simulink library "CBRModel_lib"  (Simulink 10.2)
settings: Solver=ode45  StartTime=0.0  StopTime=10.0  RelTol=1e-3  EnableMultiTasking=on
libraries: ExampleModel_lib x18, powerlib x11, $bdroot x4, powerlib_extras x4
settings Model: RequirementInfo="{}  %GIDa_6317c1c3_1285_46a1_a401_c249d430af69"  Creator=jde1  LastModifiedBy=albert

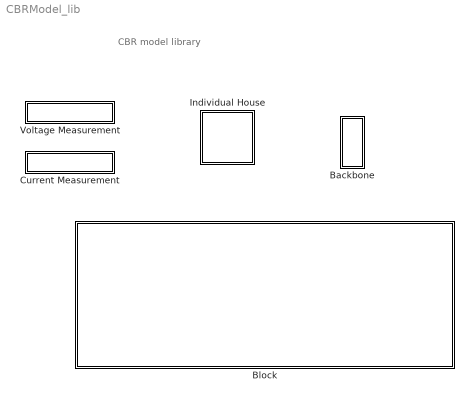
== system CBRModel_lib ==
  note: CBR model library
  Backbone : Subsystem  mask{length=0.0465}
      mask TypeOptions length: line_A/Length | line_B/Length | line_C/Length | line_N/Length
  Block : Subsystem
  Current Measurement : Subsystem  StopFcn=|
      | myname = getfullname(gcb);                                                                      
      | rto = get_param([myname '/RMS Display'], 'RuntimeObject');                                      
      | set_param(myname, 'MaskDisplay', ['color(''blue''); disp(' num2str(rto.InputPort(1).Data) ')']);
      mask Display:
      | port_label('lconn', 1, '+')
      | port_label('rconn', 1, '-')
      | color('blue')
      | disp('0')
  Individual House : Subsystem  mask{length=0.025}
      mask prompts: length "Length of service line (km)"
      mask TypeOptions length: Service Active/Length | Service Neutral/Length
      mask Display:
      | plot([20 30 40 20 20 40 40], [30 40 30 30 10 10 30])
      | port_label('LConn',1,'+')
      | port_label('RConn',1,'-')
  Voltage Measurement : Subsystem  StopFcn=|
      | myname = getfullname(gcb);                                                                      
      | rto = get_param([myname '/RMS Display'], 'RuntimeObject');                                      
      | set_param(myname, 'MaskDisplay', ['color(''blue''); disp(' num2str(rto.InputPort(1).Data) ')']);
      mask Display:
      | port_label('lconn', 1, '+')
      | port_label('rconn', 1, '-')
      | color('blue')
      | disp('0')

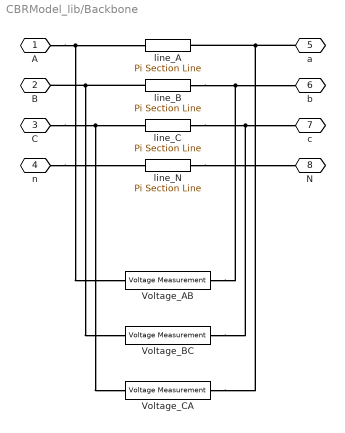
== system CBRModel_lib/Backbone ==
  Voltage_AB : $bdroot/Voltage Measurement  SystemSampleTime=-1  VariantActivationTime=update diagram  Latency=0  AutoFrameSizeCalculation=off
  Voltage_BC : $bdroot/Voltage Measurement  SystemSampleTime=-1  VariantActivationTime=update diagram  Latency=0  AutoFrameSizeCalculation=off
  Voltage_CA : $bdroot/Voltage Measurement  SystemSampleTime=-1  VariantActivationTime=update diagram  Latency=0  AutoFrameSizeCalculation=off
  line_A : powerlib/Elements/Pi Section Line  LConnTagsString=__new0  RConnTagsString=__new0  Phases=1  PiSections=1  Length=length  Frequency=50  Resistance=0.497  Inductance=1.2032e-3  Capacitance=1e-9  Measurements=None  Measurements2=None
      settings: AttributesFormatString=\n  SourceProductBaseCode=PS
  line_B : powerlib/Elements/Pi Section Line  LConnTagsString=__new0  RConnTagsString=__new0  Phases=1  PiSections=1  Length=length  Frequency=50  Resistance=0.497  Inductance=1.2032e-3  Capacitance=1e-9  Measurements=None  Measurements2=None
      settings: AttributesFormatString=\n  SourceProductBaseCode=PS
  line_C : powerlib/Elements/Pi Section Line  LConnTagsString=__new0  RConnTagsString=__new0  Phases=1  PiSections=1  Length=length  Frequency=50  Resistance=0.497  Inductance=1.2032e-3  Capacitance=1e-9  Measurements=None  Measurements2=None
      settings: AttributesFormatString=\n  SourceProductBaseCode=PS
  line_N : powerlib/Elements/Pi Section Line  LConnTagsString=__new0  RConnTagsString=__new0  Phases=1  PiSections=1  Length=length  Frequency=50  Resistance=0.497  Inductance=1.2032e-3  Capacitance=1e-9  Measurements=None  Measurements2=None
      settings: AttributesFormatString=\n  SourceProductBaseCode=PS
  A : PMIOPort  Side=Left
  B : PMIOPort  Port=2  Side=Left
  C : PMIOPort  Port=3  Side=Left
  n : PMIOPort  Port=4  Side=Left
  a : PMIOPort  Port=5  Side=Right
  b : PMIOPort  Port=6  Side=Right
  c : PMIOPort  Port=7  Side=Right
  N : PMIOPort  Port=8  Side=Right
  connections:
  n/RConn1 -- line_N/RConn1
  line_N/LConn1 -- N/RConn1
  a/RConn1 -- line_A/RConn1 -- Voltage_CA/RConn1
  line_B/RConn1 -- b/RConn1 -- Voltage_AB/RConn1
  line_C/RConn1 -- c/RConn1 -- Voltage_BC/RConn1
  C/RConn1 -- line_C/LConn1 -- Voltage_CA/LConn1
  line_B/LConn1 -- B/RConn1 -- Voltage_BC/LConn1
  A/RConn1 -- line_A/LConn1 -- Voltage_AB/LConn1

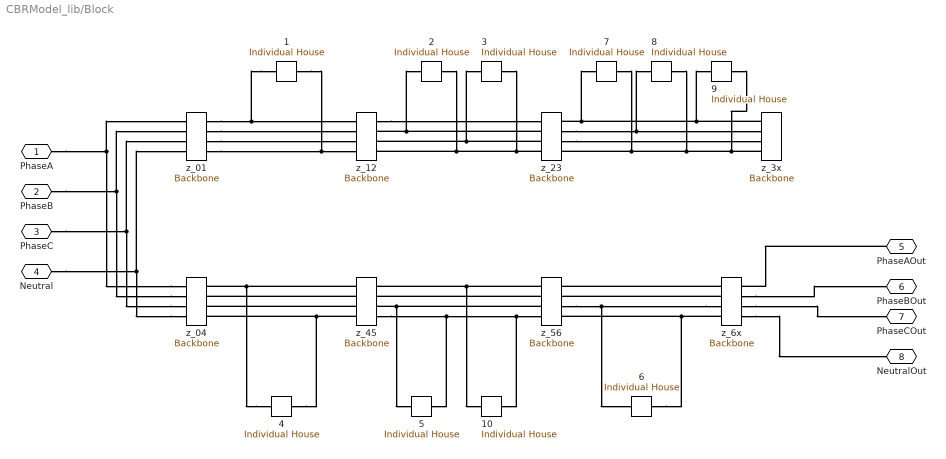
== system CBRModel_lib/Block ==
  {1..10} (10 alike) : ExampleModel_lib/Individual House  length=0.025
  z_01 : ExampleModel_lib/Backbone  length=0.02
  z_04 : ExampleModel_lib/Backbone  length=0.02
  z_{12,23,45,56} (4 alike) : ExampleModel_lib/Backbone  length=0.02
  z_3x : ExampleModel_lib/Backbone  length=0.02
  z_6x : ExampleModel_lib/Backbone  length=0.02
  PhaseA : PMIOPort  Side=Left
  PhaseB : PMIOPort  Port=2  Side=Left
  PhaseC : PMIOPort  Port=3  Side=Left
  Neutral : PMIOPort  Port=4  Side=Left
  PhaseAOut : PMIOPort  Port=5  Side=Right
  PhaseBOut : PMIOPort  Port=6  Side=Right
  PhaseCOut : PMIOPort  Port=7  Side=Right
  NeutralOut : PMIOPort  Port=8  Side=Right
  connections:
  3/LConn1 -- z_23/LConn3 -- z_12/RConn3
  10/RConn1 -- z_45/RConn4 -- 5/RConn1 -- z_56/LConn4
  z_04/LConn3 -- PhaseC/RConn1 -- z_01/LConn3
  z_04/LConn2 -- PhaseB/RConn1 -- z_01/LConn2
  7/RConn1 -- z_3x/LConn4 -- 9/RConn1 -- 8/RConn1 -- z_23/RConn4
  8/LConn1 -- z_23/RConn2 -- z_3x/LConn2
  2/RConn1 -- z_23/LConn4 -- 3/RConn1 -- z_12/RConn4
  4/RConn1 -- z_45/LConn4 -- z_04/RConn4
  7/LConn1 -- z_3x/LConn1 -- 9/LConn1 -- z_23/RConn1
  10/LConn1 -- z_56/LConn1 -- z_45/RConn1
  1/RConn1 -- z_12/LConn4 -- z_01/RConn4
  z_6x/LConn4 -- z_56/RConn4 -- 6/RConn1
  z_6x/LConn3 -- z_56/RConn3 -- 6/LConn1
  z_04/LConn1 -- PhaseA/RConn1 -- z_01/LConn1
  1/LConn1 -- z_12/LConn1 -- z_01/RConn1
  4/LConn1 -- z_45/LConn1 -- z_04/RConn1
  z_04/LConn4 -- Neutral/RConn1 -- z_01/LConn4
  5/LConn1 -- z_56/LConn3 -- z_45/RConn3
  2/LConn1 -- z_23/LConn2 -- z_12/RConn2
  PhaseAOut/RConn1 -- z_6x/RConn1
  z_56/LConn2 -- z_45/RConn2
  z_45/LConn2 -- z_04/RConn2
  z_01/RConn2 -- z_12/LConn2
  z_45/LConn3 -- z_04/RConn3
  z_6x/LConn1 -- z_56/RConn1
  z_01/RConn3 -- z_12/LConn3
  z_12/RConn1 -- z_23/LConn1
  z_23/RConn3 -- z_3x/LConn3
  z_6x/LConn2 -- z_56/RConn2
  z_6x/RConn4 -- NeutralOut/RConn1
  z_6x/RConn2 -- PhaseBOut/RConn1
  z_6x/RConn3 -- PhaseCOut/RConn1

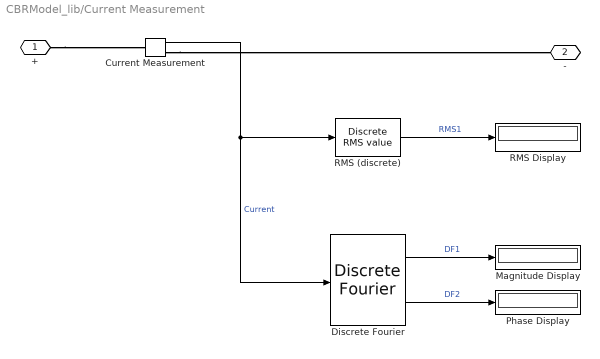
== system CBRModel_lib/Current Measurement ==
  Current Measurement : powerlib/Measurements/Current Measurement  PhasorSimulation=off  OutputType=Complex  PSBequivalent=0
  Discrete Fourier : powerlib_extras/Discrete Measurements/Discrete  Fourier  Freq=50  n=1  Par_Init=[0 0]  Ts=0.001
      settings: SourceProductBaseCode=PS
  Magnitude Display : Display
  Phase Display : Display
  RMS (discrete) : powerlib_extras/Discrete Measurements/Discrete  RMS value  Freq=50  Mag_Init=0  Ts=0.001
      settings: SourceProductBaseCode=PS
  RMS Display : Display
  + : PMIOPort  Side=Left
  - : PMIOPort  Port=2  Side=Right
  wires:
  RMS (discrete)/1 -> RMS Display/1  "RMS1"
  Discrete Fourier/1 -> Magnitude Display/1  "DF1"
  Discrete Fourier/2 -> Phase Display/1  "DF2"
  Current Measurement/1 -> Discrete Fourier/1, RMS (discrete)/1  "Current"
  connections:
  +/RConn1 -- Current Measurement/LConn1
  Current Measurement/RConn1 -- -/RConn1

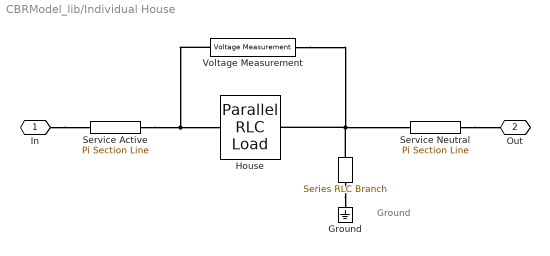
== system CBRModel_lib/Individual House ==
  note: Ground
  " " : powerlib/Elements/Series RLC Branch  LConnTagsString=__new0  RConnTagsString=__new0  BranchType=R  Resistance=10  Inductance=1e-3  SetiL0=off  InitialCurrent=0  Capacitance=1e-6  Setx0=off  InitialVoltage=0  Measurements=None
  Ground : powerlib/Elements/Ground  LConnTagsString=a
  House : powerlib/Elements/Parallel RLC Load  LConnTagsString=a  RConnTagsString=__new0  NominalVoltage=230  NominalFrequency=50  ActivePower=731.733  InductivePower=104.266  CapacitivePower=1e-06  Setx0=off  InitialVoltage=0  SetiL0=off  InitialCurrent=0  Measurements=None  LoadType=constant Z
      settings: AttributesFormatString=\n  SourceProductBaseCode=PS
  Service Active : powerlib/Elements/Pi Section Line  LConnTagsString=__new0  RConnTagsString=__new0  Phases=1  PiSections=1  Length=length  Frequency=50  Resistance=2.33  Inductance=2.833e-4  Capacitance=1e-9  Measurements=None  Measurements2=None
      settings: AttributesFormatString=\n  SourceProductBaseCode=PS
  Service Neutral : powerlib/Elements/Pi Section Line  LConnTagsString=__new0  RConnTagsString=__new0  Phases=1  PiSections=1  Length=length  Frequency=50  Resistance=2.33  Inductance=2.833e-4  Capacitance=1e-9  Measurements=None  Measurements2=None
      settings: AttributesFormatString=\n  SourceProductBaseCode=PS
  Voltage Measurement : $bdroot/Voltage Measurement  SystemSampleTime=-1  VariantActivationTime=update diagram  Latency=0  AutoFrameSizeCalculation=off
  In : PMIOPort  Side=Left
  Out : PMIOPort  Port=2  Side=Right
  connections:
  Voltage Measurement/LConn1 -- House/LConn1 -- Service Active/RConn1
  " "/RConn1 -- Ground/LConn1
  " "/LConn1 -- House/RConn1 -- Voltage Measurement/RConn1 -- Service Neutral/LConn1
  In/RConn1 -- Service Active/LConn1
  Service Neutral/RConn1 -- Out/RConn1

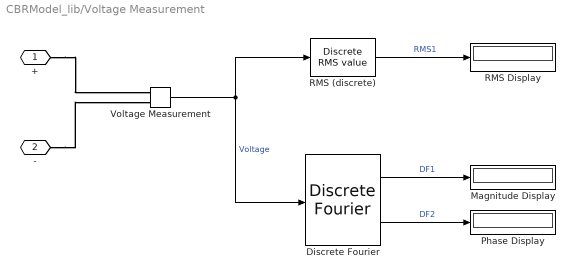
== system CBRModel_lib/Voltage Measurement ==
  Discrete Fourier : powerlib_extras/Discrete Measurements/Discrete  Fourier  Freq=50  n=1  Par_Init=[0 0]  Ts=0.001
      settings: SourceProductBaseCode=PS
  Magnitude Display : Display
  Phase Display : Display
  RMS (discrete) : powerlib_extras/Discrete Measurements/Discrete  RMS value  Freq=50  Mag_Init=0  Ts=0.001
      settings: SourceProductBaseCode=PS
  RMS Display : Display
  Voltage Measurement : powerlib/Measurements/Voltage Measurement  PhasorSimulation=off  OutputType=Complex  PSBequivalent=0
  + : PMIOPort  Side=Left
  - : PMIOPort  Port=2  Side=Right
  wires:
  Voltage Measurement/1 -> Discrete Fourier/1, RMS (discrete)/1  "Voltage"
  RMS (discrete)/1 -> RMS Display/1  "RMS1"
  Discrete Fourier/1 -> Magnitude Display/1  "DF1"
  Discrete Fourier/2 -> Phase Display/1  "DF2"
  connections:
  +/RConn1 -- Voltage Measurement/LConn1
  -/RConn1 -- Voltage Measurement/LConn2
